simulink library "Muscles4SimScienceAB"  (R2021b)
settings: Solver=VariableStepAuto  StartTime=0.0  StopTime=10.0  RelTol=1e-3
values from neighbouring files (symbols this model uses):
  jcolor = [.4 1 .6]    [init_model_parameter.m]    (also in init_simple_main.m)
  lcolor = [.2 .6 1]    [init_model_parameter.m]    (also in init_simple_main.m; init_simple_model_parameter.m = [.5, .5 , .5])
  N = length(dataset.(fldnames{1}))    [create_timeseries.m]    (also in input_data.m = length(t); test_input_data.m = length(t))
undefined symbols (not defined in the file or in its folder): bodyparam, X, Y, Z
libraries: sm_lib x21, $bdroot x9, Library_mtu_simulink x4, nesl_utility x3
settings Model: Creator=Strel  LastModifiedBy=Strel

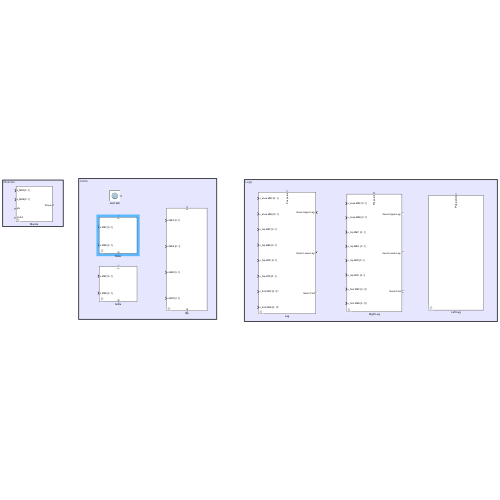
[thumbnail: Simulink's stored preview of the top-level diagram]
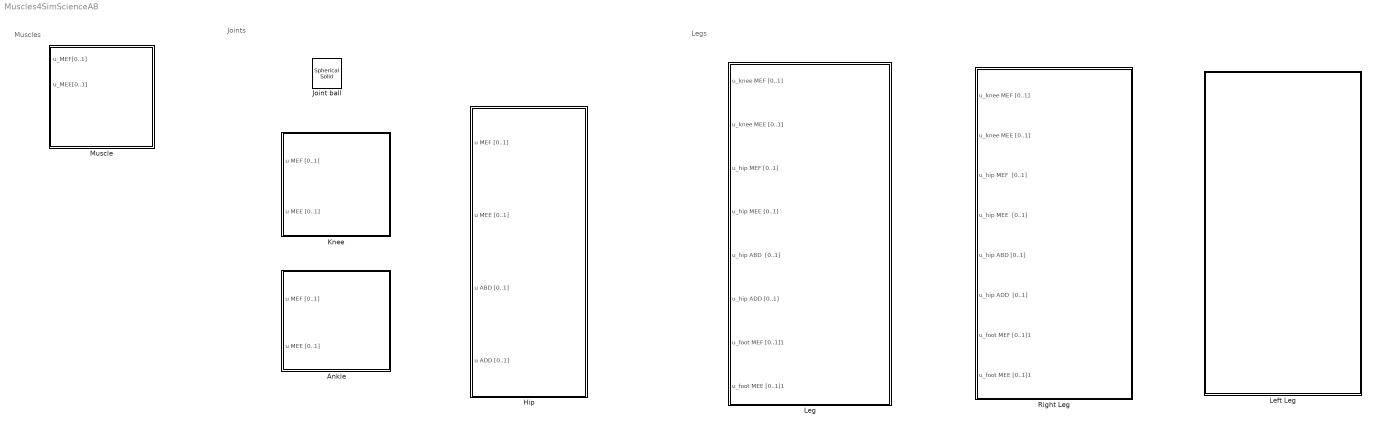
== system Muscles4SimScienceAB ==
  note: Muscles
  note: Legs
  note: Joints
  Ankle : Subsystem  mask{minlim=0, maxlim=0, stiffness=0, damping=0}
      settings: PortSchema="{\"entries\":[{\"content\":{\"sides\":[{\"content\":{\"connectorIds\":[\"In1\",\"In2\"]},\"type\":\"ConnectorPlacement.EquallySpacedRectSide\",\"uuid\":\"96b1b743-5705-4ec0-abfd-bdeea3d69127\"},{\"content\":{\"connectorIds\":[],\"side\":\"RIGHT\"},\"type\":\"ConnectorPlacement.EquallySpacedRectSide\",\"uuid\":\"b3b1b644-d2fe-42fd-b3a0-cbeacae3e2ea\"},{\"content\":{\"connectorIds\":[\"LConn1\"],\"side\":\"TOP\"},\"type\":\"ConnectorPlacement.EquallySpacedRectSide\",\"uuid\":\"6588cc9c-075c-4f00-8cf7-0671acb35c7c\"},{\"content\":{\"connectorIds\":[\"RConn1\"],\"side\":\"BOTTOM\"},\"type\":\"ConnectorPlacement.EquallySpacedRectSide\",\"uuid\":\"1f17b914-0342-4251-8355-6f738c5be59c\"}]},\"type\":\"ConnectorPlacement.EquallySpacedConnector\",\"uuid\":\"9665cf7e-0d90-4f65-9e3e-57dbf89b4304\"}],\"packageUris\":[\"http://schema.mathworks.com/mf0/Connector/R2020b\"],\"version\":\"1.0\"}"
  Hip : Subsystem  mask{minlim_x=0, maxlim_x=0, minlim_y=0, maxlim_y=0, stiffness=0, damping=0}
      settings: PortSchema="{\"entries\":[{\"content\":{\"sides\":[{\"content\":{\"connectorIds\":[\"In1\",\"In2\",\"In3\",\"In4\"]},\"type\":\"ConnectorPlacement.EquallySpacedRectSide\",\"uuid\":\"41193043-8a27-4363-8898-1f9e881d08b1\"},{\"content\":{\"connectorIds\":[],\"side\":\"RIGHT\"},\"type\":\"ConnectorPlacement.EquallySpacedRectSide\",\"uuid\":\"5a179196-4a66-423b-80c7-02c9aceed262\"},{\"content\":{\"connectorIds\":[\"LConn1\"],\"side\":\"TOP\"},\"type\":\"ConnectorPlacement.EquallySpacedRectSide\",\"uuid\":\"db447b50-73cc-4af2-8c9c-28a9801561ff\"},{\"content\":{\"connectorIds\":[\"RConn1\"],\"side\":\"BOTTOM\"},\"type\":\"ConnectorPlacement.EquallySpacedRectSide\",\"uuid\":\"bc7ed954-e11d-4420-941c-b14a31097b3c\"}]},\"type\":\"ConnectorPlacement.EquallySpacedConnector\",\"uuid\":\"a73193d2-090f-471b-ad63-2ab894437460\"}],\"packageUris\":[\"http://schema.mathworks.com/mf0/Connector/R2020b\"],\"version\":\"1.0\"}"
  Joint ball : sm_lib/Body Elements/Spherical Solid  GraphicAmbientColor=[0.15 0.15 0.15 1.0]  BasedOnType=Mass  CenterOfMass=[0 0 0]  CenterOfMassUnits=m  GraphicDiffuseColor=[1.0 1.0 0.2]  Density=1000  DensityUnits=kg/m^3  DoExposeReferenceFrame=on  GraphicEmissiveColor=[0.0 0.0 0.0 1.0]  ExportEntireGeometry=off  SerializedExposedGeometries=<ExposedGeometries/>  SerializedFrames=<Frames/>  MarkerShape=Sphere  MarkerSize=10  GraphicType=FromGeometry  InertiaType=CalculateFromGeometry  Mass=0  MassUnits=kg  MomentsOfInertia=[1 1 1]  MomentsOfInertiaUnits=kg*m^2  GraphicOpacity=1.0  ProductsOfInertia=[0 0 0]  ProductsOfInertiaUnits=kg*m^2  GraphicShininess=75  GraphicSpecularColor=[0.5 0.5 0.5 1.0]  SphereRadius=bodyparam.size.jointballs  SphereRadiusUnits=m  GraphicVisPropType=SimpleVisualProperties
  Knee : Subsystem  mask{maxlim=0, minlim=0, stiffness=0, damping=0}
      settings: PortSchema="{\"entries\":[{\"content\":{\"sides\":[{\"content\":{\"connectorIds\":[\"In1\",\"In2\"]},\"type\":\"ConnectorPlacement.EquallySpacedRectSide\",\"uuid\":\"41193043-8a27-4363-8898-1f9e881d08b1\"},{\"content\":{\"connectorIds\":[],\"side\":\"RIGHT\"},\"type\":\"ConnectorPlacement.EquallySpacedRectSide\",\"uuid\":\"5a179196-4a66-423b-80c7-02c9aceed262\"},{\"content\":{\"connectorIds\":[\"LConn1\"],\"side\":\"TOP\"},\"type\":\"ConnectorPlacement.EquallySpacedRectSide\",\"uuid\":\"db447b50-73cc-4af2-8c9c-28a9801561ff\"},{\"content\":{\"connectorIds\":[\"RConn1\"],\"side\":\"BOTTOM\"},\"type\":\"ConnectorPlacement.EquallySpacedRectSide\",\"uuid\":\"bc7ed954-e11d-4420-941c-b14a31097b3c\"}]},\"type\":\"ConnectorPlacement.EquallySpacedConnector\",\"uuid\":\"a73193d2-090f-471b-ad63-2ab894437460\"}],\"packageUris\":[\"http://schema.mathworks.com/mf0/Connector/R2020b\"],\"version\":\"1.0\"}"
  Left Leg : Subsystem  mask{pos=bodyparam.position.left, sp=bodyparam.sp.left}
      mask prompts: pos "Position"; sp "Center of Mass"
      settings: PortSchema="{\"entries\":[{\"content\":{\"sides\":[{\"content\":{\"connectorIds\":[]},\"type\":\"ConnectorPlacement.EquallySpacedRectSide\",\"uuid\":\"83ecb678-3ef8-433f-8d5c-ab0d2505f36e\"},{\"content\":{\"connectorIds\":[],\"side\":\"RIGHT\"},\"type\":\"ConnectorPlacement.EquallySpacedRectSide\",\"uuid\":\"d8e24638-d682-4ec3-8d5e-a9f0648ccc2e\"},{\"content\":{\"connectorIds\":[\"LConn1\"],\"side\":\"TOP\"},\"type\":\"ConnectorPlacement.EquallySpacedRectSide\",\"uuid\":\"3cc5390e-ac28-4512-8909-8c109732ea75\"}]},\"type\":\"ConnectorPlacement.EquallySpacedConnector\",\"uuid\":\"7489c74b-9d79-4343-b8bc-4ccd280d7c44\"}],\"packageUris\":[\"http://schema.mathworks.com/mf0/Connector/R2020b\"],\"version\":\"1.0\"}"
  Leg : Subsystem  mask{size=bodyparam.size, pos=bodyparam.position, weight=bodyparam.weight, sp=bodyparam.sp, maxlim=bodyparam.maxlim, minlim=bodyparam.minlim, stiffness=bodyparam.stiffness, damping=bodyparam.damping, jcolor=jcolor, lcolor=lcolor}
      mask prompts: pos "Position"; sp "Center of mass"; jcolor "Joint Color"; lcolor "Leg Color"
      settings: PortSchema="{\"entries\":[{\"content\":{\"sides\":[{\"content\":{\"connectorIds\":[\"In1\",\"In2\",\"In3\",\"In4\",\"In5\",\"In6\",\"In7\",\"In8\"]},\"type\":\"ConnectorPlacement.EquallySpacedRectSide\",\"uuid\":\"047c7818-584d-43bc-9ac6-0cf7022720ad\"},{\"content\":{\"connectorIds\":[\"RConn1\",\"RConn2\",\"RConn3\"],\"side\":\"RIGHT\"},\"type\":\"ConnectorPlacement.EquallySpacedRectSide\",\"uuid\":\"5ae6b5e3-6d8b-484f-b2c6-d9c9ef2af35a\"},{\"content\":{\"connectorIds\":[\"LConn1\"],\"side\":\"TOP\"},\"type\":\"ConnectorPlacement.EquallySpacedRectSide\",\"uuid\":\"10998751-961f-47ac-ace7-fed01c97684e\"}]},\"type\":\"ConnectorPlacement.EquallySpacedConnector\",\"uuid\":\"80eaa50d-578f-4e76-a7ef-cf0f1326b1e3\"}],\"packageUris\":[\"http://schema.mathworks.com/mf0/Connector/R2020b\"],\"version\":\"1.0\"}"
  Muscle : Subsystem  mask{Param_Mus_MEF=0, Param_Mus_MEE=0, r=0}
      mask prompts: r "Leverage"
  Right Leg : Subsystem  mask{pos=bodyparam.position.right, sp=bodyparam.sp.right}
      mask prompts: pos "Position"; sp "Center of Mass"
      settings: PortSchema="{\"entries\":[{\"content\":{\"sides\":[{\"content\":{\"connectorIds\":[\"In1\",\"In2\",\"In3\",\"In4\",\"In5\",\"In6\",\"In7\",\"In8\"]},\"type\":\"ConnectorPlacement.EquallySpacedRectSide\",\"uuid\":\"83ecb678-3ef8-433f-8d5c-ab0d2505f36e\"},{\"content\":{\"connectorIds\":[\"RConn1\",\"RConn2\",\"RConn3\"],\"side\":\"RIGHT\"},\"type\":\"ConnectorPlacement.EquallySpacedRectSide\",\"uuid\":\"d8e24638-d682-4ec3-8d5e-a9f0648ccc2e\"},{\"content\":{\"connectorIds\":[\"LConn1\"],\"side\":\"TOP\"},\"type\":\"ConnectorPlacement.EquallySpacedRectSide\",\"uuid\":\"3cc5390e-ac28-4512-8909-8c109732ea75\"}]},\"type\":\"ConnectorPlacement.EquallySpacedConnector\",\"uuid\":\"7489c74b-9d79-4343-b8bc-4ccd280d7c44\"}],\"packageUris\":[\"http://schema.mathworks.com/mf0/Connector/R2020b\"],\"version\":\"1.0\"}"

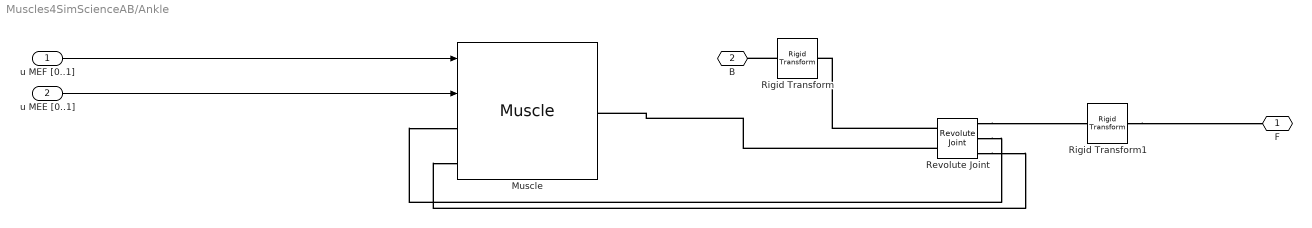
== system Muscles4SimScienceAB/Ankle ==
  u MEF [0..1] : Inport
  u MEE [0..1] : Inport  Port=2
  Muscle : $bdroot/Muscle  Param_Mus_MEF=Param_Mus_MEF_knee  Param_Mus_MEE=Param_Mus_MEE_knee  r=bodyparam.r.foot
  Revolute Joint : sm_lib/Joints/Revolute Joint  JointMode=Normal  SenseConstraintForce=off  SenseConstraintForceX=off  SenseConstraintForceY=off  SenseConstraintForceZ=off  SenseConstraintTorque=off  SenseConstraintTorqueX=off  SenseConstraintTorqueY=off  SenseConstraintTorqueZ=off  SenseTotalForce=off  SenseTotalForceX=off  SenseTotalForceY=off  SenseTotalForceZ=off  SenseTotalTorque=off  SenseTotalTorqueX=off  SenseTotalTorqueY=off  SenseTotalTorqueZ=off  CompositeWrenchDir=FollowerOnBase  CompositeWrenchFrame=BaseFrame  EquilibriumPosition=0  EquilibriumPositionUnits=deg  SpringStiffness=0  SpringStiffnessUnits=N*m/deg  DampingCoefficient=0  DampingCoefficientUnits=N*m/(deg/s)  TorqueActuationMode=InputTorque  MotionActuationMode=ComputedMotion  SensePosition=on  SenseVelocity=on  SenseAcceleration=off  SenseTorqueForce=off  SenseLowerLimitTorqueForce=off  SenseUpperLimitTorqueForce=off  LowerLimitSpecify=on  LowerLimitBound=minlim  LowerLimitBoundUnits=deg  LowerLimitStiffness=stiffness  LowerLimitStiffnessUnits=N*m/deg  LowerLimitDamping=damping  LowerLimitDampingUnits=N*m/(deg/s)  LowerLimitTransitionRegionWidth=0.1  LowerLimitTransitionRegionWidthUnits=deg  UpperLimitSpecify=on  UpperLimitBound=maxlim  UpperLimitBoundUnits=deg  UpperLimitStiffness=stiffness  UpperLimitStiffnessUnits=N*m/deg  UpperLimitDamping=damping  UpperLimitDampingUnits=N*m/(deg/s)  UpperLimitTransitionRegionWidth=0.1  UpperLimitTransitionRegionWidthUnits=deg  PositionTargetSpecify=off  PositionTargetPriority=High  PositionTargetValue=0  PositionTargetValueUnits=deg  VelocityTargetSpecify=off  VelocityTargetPriority=High  VelocityTargetValue=0  VelocityTargetValueUnits=deg/s
  Rigid Transform : sm_lib/Frames and Transforms/Rigid Transform  TranslationMethod=None  TranslationStandardOffset=0  TranslationLengthUnit=m  TranslationStandardAxis=+Z  TranslationCartesianOffset=[0 0 0]  TranslationROffset=0  TranslationROffsetUnits=m  TranslationZOffset=0  TranslationZOffsetUnits=m  TranslationThetaOffset=0  TranslationThetaOffsetUnits=deg  RotationMethod=StandardAxis  RotationAngleUnits=deg  RotationStandardAxis=+X  RotationAngle=-90  RotationArbitraryAxis=[0 0 1]  FollAlignAxisA=+X  BaseAlignAxisA=+Y  FollAlignAxisB=+Y  BaseAlignAxisB=+Z  RotationSequenceAxes=FollowerAxes  RotationSequence=XYX  RotationSequenceAngles=[0 0 0]  RotationSequenceAnglesUnits=deg  RotationMatrix=[1 0 0; 0 1 0; 0 0 1]
  Rigid Transform1 : sm_lib/Frames and Transforms/Rigid Transform  TranslationMethod=None  TranslationStandardOffset=0  TranslationLengthUnit=m  TranslationStandardAxis=+Z  TranslationCartesianOffset=[0 0 0]  TranslationROffset=0  TranslationROffsetUnits=m  TranslationZOffset=0  TranslationZOffsetUnits=m  TranslationThetaOffset=0  TranslationThetaOffsetUnits=deg  RotationMethod=StandardAxis  RotationAngleUnits=deg  RotationStandardAxis=+X  RotationAngle=90  RotationArbitraryAxis=[0 0 1]  FollAlignAxisA=+X  BaseAlignAxisA=+Y  FollAlignAxisB=+Y  BaseAlignAxisB=+Z  RotationSequenceAxes=FollowerAxes  RotationSequence=XYX  RotationSequenceAngles=[0 0 0]  RotationSequenceAnglesUnits=deg  RotationMatrix=[1 0 0; 0 1 0; 0 0 1]
  F : PMIOPort  Side=Left
  B : PMIOPort  Port=2  Side=Right
  wires:
  u MEE [0..1]/1 -> Muscle/2
  u MEF [0..1]/1 -> Muscle/1
  connections:
  Rigid Transform/LConn1 -- B/RConn1
  Revolute Joint/RConn1 -- Rigid Transform1/LConn1
  Revolute Joint/LConn2 -- Muscle/RConn1
  Revolute Joint/RConn3 -- Muscle/LConn2
  Revolute Joint/LConn1 -- Rigid Transform/RConn1
  Rigid Transform1/RConn1 -- F/RConn1
  Revolute Joint/RConn2 -- Muscle/LConn1

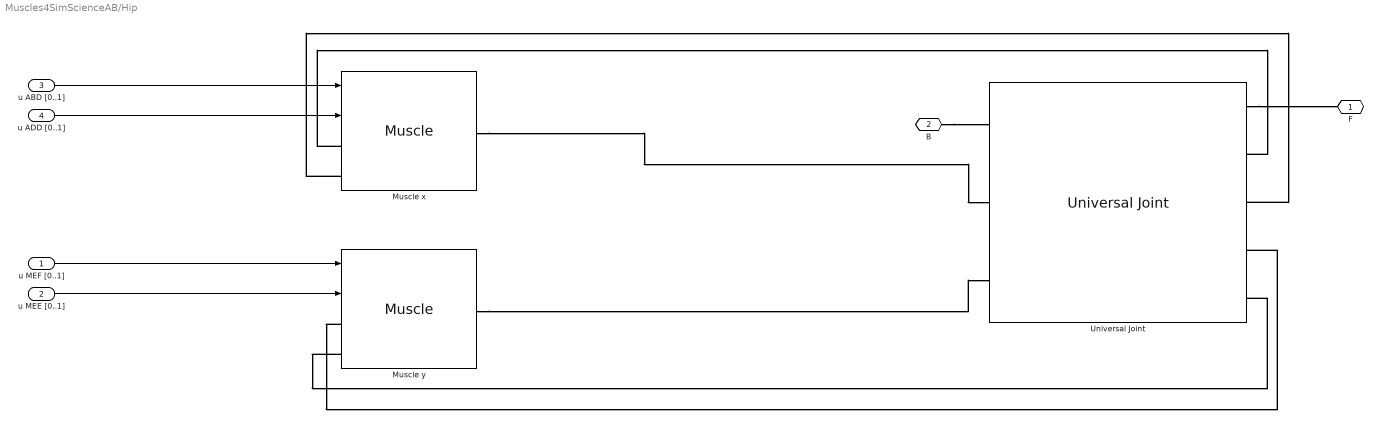
== system Muscles4SimScienceAB/Hip ==
  u MEF [0..1] : Inport
  u MEE [0..1] : Inport  Port=2
  u ABD [0..1] : Inport  Port=3
  u ADD [0..1] : Inport  Port=4
  Muscle x : $bdroot/Muscle  Param_Mus_MEF=Param_Mus_MEF_hip  Param_Mus_MEE=Param_Mus_MEE_hip  r=bodyparam.r.hip.ef
  Muscle y : $bdroot/Muscle  Param_Mus_MEF=Param_Mus_ABD_hip  Param_Mus_MEE=Param_Mus_ADD_hip  r=bodyparam.r.hip.abd
  Universal Joint : sm_lib/Joints/Universal Joint  JointMode=Normal  SenseConstraintForce=off  SenseConstraintForceX=off  SenseConstraintForceY=off  SenseConstraintForceZ=off  SenseConstraintTorque=off  SenseConstraintTorqueX=off  SenseConstraintTorqueY=off  SenseConstraintTorqueZ=off  SenseTotalForce=off  SenseTotalForceX=off  SenseTotalForceY=off  SenseTotalForceZ=off  SenseTotalTorque=off  SenseTotalTorqueX=off  SenseTotalTorqueY=off  SenseTotalTorqueZ=off  CompositeWrenchDir=FollowerOnBase  CompositeWrenchFrame=BaseFrame  RxEquilibriumPosition=0  RxEquilibriumPositionUnits=deg  RxSpringStiffness=0  RxSpringStiffnessUnits=N*m/deg  RxDampingCoefficient=0  RxDampingCoefficientUnits=N*m/(deg/s)  RxTorqueActuationMode=InputTorque  RxMotionActuationMode=ComputedMotion  RxSensePosition=on  RxSenseVelocity=on  RxSenseAcceleration=off  RxSenseTorqueForce=off  RxSenseLowerLimitTorqueForce=off  RxSenseUpperLimitTorqueForce=off  RxLowerLimitSpecify=on  RxLowerLimitBound=minlim_x  RxLowerLimitBoundUnits=deg  RxLowerLimitStiffness=stiffness  RxLowerLimitStiffnessUnits=N*m/deg  RxLowerLimitDamping=damping  RxLowerLimitDampingUnits=N*m/(deg/s)  RxLowerLimitTransitionRegionWidth=0.1  RxLowerLimitTransitionRegionWidthUnits=deg  RxUpperLimitSpecify=on  RxUpperLimitBound=maxlim_x  RxUpperLimitBoundUnits=deg  RxUpperLimitStiffness=stiffness  RxUpperLimitStiffnessUnits=N*m/deg  RxUpperLimitDamping=damping  RxUpperLimitDampingUnits=N*m*s/deg  RxUpperLimitTransitionRegionWidth=0.1  RxUpperLimitTransitionRegionWidthUnits=deg  RxPositionTargetSpecify=off  RxPositionTargetPriority=High  RxPositionTargetValue=0  RxPositionTargetValueUnits=deg  RxVelocityTargetSpecify=off  RxVelocityTargetPriority=High  RxVelocityTargetValue=0  RxVelocityTargetValueUnits=deg/s  RyEquilibriumPosition=0  RyEquilibriumPositionUnits=deg  RySpringStiffness=0  RySpringStiffnessUnits=N*m/deg  RyDampingCoefficient=0  RyDampingCoefficientUnits=N*m/(deg/s)  RyTorqueActuationMode=InputTorque  RyMotionActuationMode=ComputedMotion  RySensePosition=on  RySenseVelocity=on  RySenseAcceleration=off  RySenseTorqueForce=off  RySenseLowerLimitTorqueForce=off  RySenseUpperLimitTorqueForce=off  RyLowerLimitSpecify=on  RyLowerLimitBound=minlim_y  RyLowerLimitBoundUnits=deg  RyLowerLimitStiffness=stiffness  RyLowerLimitStiffnessUnits=N*m/deg  RyLowerLimitDamping=damping  RyLowerLimitDampingUnits=N*m/(deg/s)  RyLowerLimitTransitionRegionWidth=0.1  RyLowerLimitTransitionRegionWidthUnits=deg  RyUpperLimitSpecify=on  RyUpperLimitBound=maxlim_y  RyUpperLimitBoundUnits=deg  RyUpperLimitStiffness=stiffness  RyUpperLimitStiffnessUnits=N*m/deg  RyUpperLimitDamping=damping  RyUpperLimitDampingUnits=N*m/(deg/s)  RyUpperLimitTransitionRegionWidth=0.1  RyUpperLimitTransitionRegionWidthUnits=deg  RyPositionTargetSpecify=off  RyPositionTargetPriority=High  RyPositionTargetValue=0  RyPositionTargetValueUnits=deg  RyVelocityTargetSpecify=off  RyVelocityTargetPriority=High  RyVelocityTargetValue=0  RyVelocityTargetValueUnits=deg/s
  F : PMIOPort  Side=Left
  B : PMIOPort  Port=2  Side=Right
  wires:
  u ABD [0..1]/1 -> Muscle x/1
  u ADD [0..1]/1 -> Muscle x/2
  u MEF [0..1]/1 -> Muscle y/1
  u MEE [0..1]/1 -> Muscle y/2
  connections:
  Muscle x/RConn1 -- Universal Joint/LConn2
  Muscle y/RConn1 -- Universal Joint/LConn3
  B/RConn1 -- Universal Joint/LConn1
  Muscle x/LConn1 -- Universal Joint/RConn2
  Universal Joint/RConn1 -- F/RConn1
  Muscle x/LConn2 -- Universal Joint/RConn3
  Muscle y/LConn1 -- Universal Joint/RConn4
  Muscle y/LConn2 -- Universal Joint/RConn5

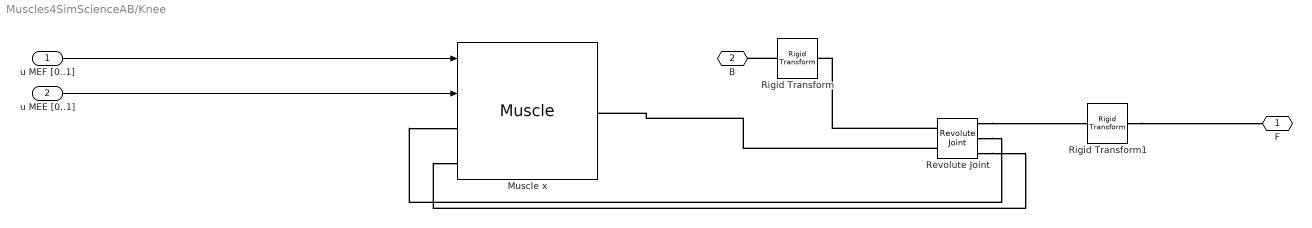
== system Muscles4SimScienceAB/Knee ==
  u MEF [0..1] : Inport
  u MEE [0..1] : Inport  Port=2
  Muscle x : $bdroot/Muscle  Param_Mus_MEF=Param_Mus_MEF_knee  Param_Mus_MEE=Param_Mus_MEE_knee  r=bodyparam.r.knee
  Revolute Joint : sm_lib/Joints/Revolute Joint  JointMode=Normal  SenseConstraintForce=off  SenseConstraintForceX=off  SenseConstraintForceY=off  SenseConstraintForceZ=off  SenseConstraintTorque=off  SenseConstraintTorqueX=off  SenseConstraintTorqueY=off  SenseConstraintTorqueZ=off  SenseTotalForce=off  SenseTotalForceX=off  SenseTotalForceY=off  SenseTotalForceZ=off  SenseTotalTorque=off  SenseTotalTorqueX=off  SenseTotalTorqueY=off  SenseTotalTorqueZ=off  CompositeWrenchDir=FollowerOnBase  CompositeWrenchFrame=BaseFrame  EquilibriumPosition=0  EquilibriumPositionUnits=deg  SpringStiffness=0  SpringStiffnessUnits=N*m/deg  DampingCoefficient=0  DampingCoefficientUnits=N*m/(deg/s)  TorqueActuationMode=InputTorque  MotionActuationMode=ComputedMotion  SensePosition=on  SenseVelocity=on  SenseAcceleration=off  SenseTorqueForce=off  SenseLowerLimitTorqueForce=off  SenseUpperLimitTorqueForce=off  LowerLimitSpecify=on  LowerLimitBound=minlim  LowerLimitBoundUnits=deg  LowerLimitStiffness=stiffness  LowerLimitStiffnessUnits=N*m/deg  LowerLimitDamping=damping  LowerLimitDampingUnits=N*m/(deg/s)  LowerLimitTransitionRegionWidth=0.1  LowerLimitTransitionRegionWidthUnits=deg  UpperLimitSpecify=on  UpperLimitBound=maxlim  UpperLimitBoundUnits=deg  UpperLimitStiffness=stiffness  UpperLimitStiffnessUnits=N*m/deg  UpperLimitDamping=damping  UpperLimitDampingUnits=N*m/(deg/s)  UpperLimitTransitionRegionWidth=0.1  UpperLimitTransitionRegionWidthUnits=deg  PositionTargetSpecify=off  PositionTargetPriority=High  PositionTargetValue=0  PositionTargetValueUnits=deg  VelocityTargetSpecify=off  VelocityTargetPriority=High  VelocityTargetValue=0  VelocityTargetValueUnits=deg/s
  Rigid Transform : sm_lib/Frames and Transforms/Rigid Transform  TranslationMethod=None  TranslationStandardOffset=0  TranslationLengthUnit=m  TranslationStandardAxis=+Z  TranslationCartesianOffset=[0 0 0]  TranslationROffset=0  TranslationROffsetUnits=m  TranslationZOffset=0  TranslationZOffsetUnits=m  TranslationThetaOffset=0  TranslationThetaOffsetUnits=deg  RotationMethod=StandardAxis  RotationAngleUnits=deg  RotationStandardAxis=+X  RotationAngle=-90  RotationArbitraryAxis=[0 0 1]  FollAlignAxisA=+X  BaseAlignAxisA=+Y  FollAlignAxisB=+Y  BaseAlignAxisB=+Z  RotationSequenceAxes=FollowerAxes  RotationSequence=XYX  RotationSequenceAngles=[0 0 0]  RotationSequenceAnglesUnits=deg  RotationMatrix=[1 0 0; 0 1 0; 0 0 1]
  Rigid Transform1 : sm_lib/Frames and Transforms/Rigid Transform  TranslationMethod=None  TranslationStandardOffset=0  TranslationLengthUnit=m  TranslationStandardAxis=+Z  TranslationCartesianOffset=[0 0 0]  TranslationROffset=0  TranslationROffsetUnits=m  TranslationZOffset=0  TranslationZOffsetUnits=m  TranslationThetaOffset=0  TranslationThetaOffsetUnits=deg  RotationMethod=StandardAxis  RotationAngleUnits=deg  RotationStandardAxis=+X  RotationAngle=90  RotationArbitraryAxis=[0 0 1]  FollAlignAxisA=+X  BaseAlignAxisA=+Y  FollAlignAxisB=+Y  BaseAlignAxisB=+Z  RotationSequenceAxes=FollowerAxes  RotationSequence=XYX  RotationSequenceAngles=[0 0 0]  RotationSequenceAnglesUnits=deg  RotationMatrix=[1 0 0; 0 1 0; 0 0 1]
  F : PMIOPort  Side=Left
  B : PMIOPort  Port=2  Side=Right
  wires:
  u MEE [0..1]/1 -> Muscle x/2
  u MEF [0..1]/1 -> Muscle x/1
  connections:
  Revolute Joint/LConn1 -- Rigid Transform/RConn1
  Revolute Joint/LConn2 -- Muscle x/RConn1
  Rigid Transform1/RConn1 -- F/RConn1
  Revolute Joint/RConn2 -- Muscle x/LConn1
  Revolute Joint/RConn3 -- Muscle x/LConn2
  Rigid Transform/LConn1 -- B/RConn1
  Revolute Joint/RConn1 -- Rigid Transform1/LConn1

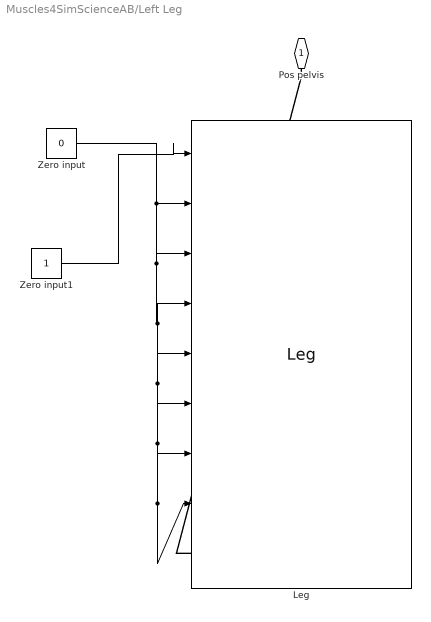
== system Muscles4SimScienceAB/Left Leg ==
  Leg : $bdroot/Leg  size=bodyparam.size  pos=pos  weight=bodyparam.weight  sp=sp  maxlim=bodyparam.maxlim  minlim=bodyparam.minlim  stiffness=bodyparam.stiffness  damping=bodyparam.damping  jcolor=jcolor  lcolor=lcolor
      link override Upper Leg Right/Hip: minlim_x=minlim.hip.ef  maxlim_x=maxlim.hip.ef  minlim_y=minlim.hip.abd  maxlim_y=maxlim.hip.abd  stiffness=stiffness.hip  damping=damping.hip
  Zero input : Constant  Value=0
  Zero input1 : Constant
  Pos pelvis : PMIOPort  Side=Left
  wires:
  Zero input/1 -> Leg/2, Leg/3, Leg/4, Leg/5, Leg/6, Leg/7, Leg/8
  Zero input1/1 -> Leg/1
  connections:
  Leg/LConn1 -- Pos pelvis/RConn1

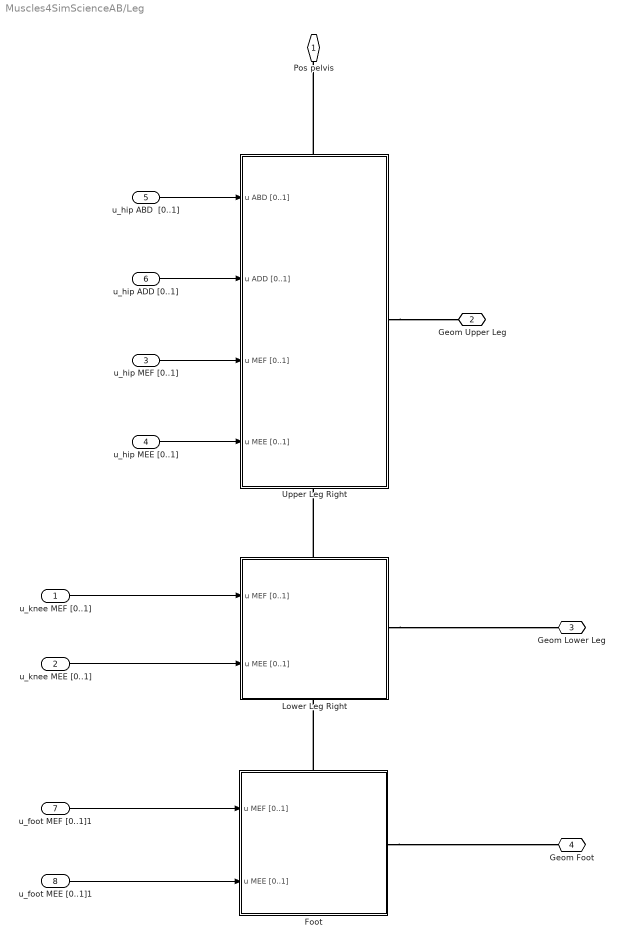
== system Muscles4SimScienceAB/Leg ==
  u_knee MEF [0..1] : Inport
  u_knee MEE [0..1] : Inport  Port=2
  u_hip MEF [0..1] : Inport  Port=3
  u_hip MEE [0..1] : Inport  Port=4
  u_hip ABD  [0..1] : Inport  Port=5
  u_hip ADD [0..1] : Inport  Port=6
  u_foot MEF [0..1]1 : Inport  Port=7
  u_foot MEE [0..1]1 : Inport  Port=8
  Foot : Subsystem
      settings: PortSchema="{\"entries\":[{\"content\":{\"sides\":[{\"content\":{\"connectorIds\":[]},\"type\":\"ConnectorPlacement.EquallySpacedRectSide\",\"uuid\":\"d033d68b-6c1a-4130-88bc-96923c9206ae\"},{\"content\":{\"connectorIds\":[\"RConn1\"],\"side\":\"RIGHT\"},\"type\":\"ConnectorPlacement.EquallySpacedRectSide\",\"uuid\":\"aebe2891-e167-481b-874d-322841d1d85d\"},{\"content\":{\"connectorIds\":[\"In1\",\"In2\"],\"side\":\"TOP\"},\"type\":\"ConnectorPlacement.EquallySpacedRectSide\",\"uuid\":\"02ffbb51-7d33-4a0b-abb1-a48a3de38eb7\"},{\"content\":{\"connectorIds\":[\"RConn2\"],\"side\":\"BOTTOM\"},\"type\":\"ConnectorPlacement.EquallySpacedRectSide\",\"uuid\":\"55de7e85-58cc-4707-ad35-b95b4479c51b\"}]},\"type\":\"ConnectorPlacement.EquallySpacedConnector\",\"uuid\":\"eef9a049-18d9-4a2f-a245-6d7e22390965\"}],\"packageUris\":[\"http://schema.mathworks.com/mf0/Connector/R2020b\"],\"version\":\"1.0\"}"
  Lower Leg Right : Subsystem
      settings: PortSchema="{\"entries\":[{\"content\":{\"sides\":[{\"content\":{\"connectorIds\":[\"LConn1\"]},\"type\":\"ConnectorPlacement.EquallySpacedRectSide\",\"uuid\":\"81fd97e6-5a65-4706-89fa-4293b691d4da\"},{\"content\":{\"connectorIds\":[\"RConn1\"],\"side\":\"RIGHT\"},\"type\":\"ConnectorPlacement.EquallySpacedRectSide\",\"uuid\":\"97541aff-136c-4e86-8809-6e6381c3329c\"},{\"content\":{\"connectorIds\":[\"In1\",\"In2\"],\"side\":\"TOP\"},\"type\":\"ConnectorPlacement.EquallySpacedRectSide\",\"uuid\":\"ce41e290-bfc8-4dfc-8c5e-525607ac3665\"},{\"content\":{\"connectorIds\":[\"RConn2\"],\"side\":\"BOTTOM\"},\"type\":\"ConnectorPlacement.EquallySpacedRectSide\",\"uuid\":\"f37d3c0f-447d-4b24-96cc-929e66a7279d\"}]},\"type\":\"ConnectorPlacement.EquallySpacedConnector\",\"uuid\":\"c782017f-7d61-4987-8163-b5d1e1eaf397\"}],\"packageUris\":[\"http://schema.mathworks.com/mf0/Connector/R2020b\"],\"version\":\"1.0\"}"
  Upper Leg Right : Subsystem
      settings: PortSchema="{\"entries\":[{\"content\":{\"sides\":[{\"content\":{\"connectorIds\":[\"LConn1\"]},\"type\":\"ConnectorPlacement.EquallySpacedRectSide\",\"uuid\":\"81fd97e6-5a65-4706-89fa-4293b691d4da\"},{\"content\":{\"connectorIds\":[\"RConn1\"],\"side\":\"RIGHT\"},\"type\":\"ConnectorPlacement.EquallySpacedRectSide\",\"uuid\":\"97541aff-136c-4e86-8809-6e6381c3329c\"},{\"content\":{\"connectorIds\":[\"In1\",\"In2\",\"In3\",\"In4\"],\"side\":\"TOP\"},\"type\":\"ConnectorPlacement.EquallySpacedRectSide\",\"uuid\":\"ce41e290-bfc8-4dfc-8c5e-525607ac3665\"},{\"content\":{\"connectorIds\":[\"RConn2\"],\"side\":\"BOTTOM\"},\"type\":\"ConnectorPlacement.EquallySpacedRectSide\",\"uuid\":\"2db09f85-d22e-4c52-ab8b-45b3630dfd34\"}]},\"type\":\"ConnectorPlacement.EquallySpacedConnector\",\"uuid\":\"c782017f-7d61-4987-8163-b5d1e1eaf397\"}],\"packageUris\":[\"http://schema.mathworks.com/mf0/Connector/R2020b\"],\"version\":\"1.0\"}"
  Pos pelvis : PMIOPort  Side=Left
  "Geom Upper Leg " : PMIOPort  Port=2  Side=Right
  "Geom Lower Leg " : PMIOPort  Port=3  Side=Right
  Geom Foot : PMIOPort  Port=4  Side=Right
  wires:
  u_knee MEF [0..1]/1 -> Lower Leg Right/2(u MEF [0..1])
  u_knee MEE [0..1]/1 -> Lower Leg Right/1(u MEE [0..1])
  u_foot MEF [0..1]1/1 -> Foot/2(u MEF [0..1])
  u_foot MEE [0..1]1/1 -> Foot/1(u MEE [0..1])
  u_hip ADD [0..1]/1 -> Upper Leg Right/3(u ADD [0..1])
  u_hip ABD  [0..1]/1 -> Upper Leg Right/4(u ABD [0..1])
  u_hip MEF [0..1]/1 -> Upper Leg Right/2(u MEF [0..1])
  u_hip MEE [0..1]/1 -> Upper Leg Right/1(u MEE [0..1])
  connections:
  Upper Leg Right/RConn1 -- Pos pelvis/RConn1
  Upper Leg Right/RConn2 -- "Geom Upper Leg "/RConn1
  Foot/RConn1 -- Lower Leg Right/LConn1
  Lower Leg Right/RConn2 -- "Geom Lower Leg "/RConn1
  Lower Leg Right/RConn1 -- Upper Leg Right/LConn1
  Foot/RConn2 -- Geom Foot/RConn1

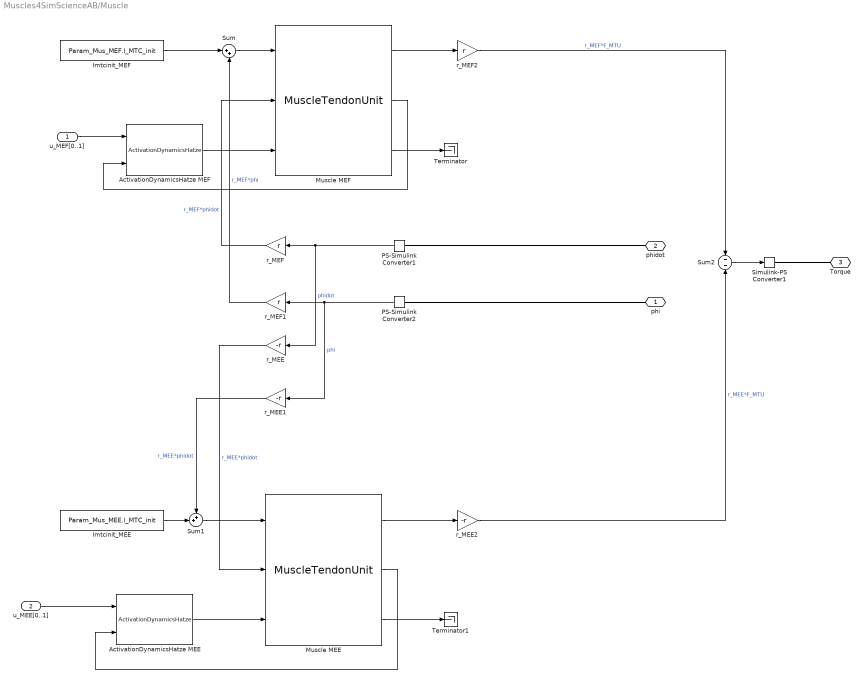
== system Muscles4SimScienceAB/Muscle ==
  u_MEF[0..1] : Inport
  u_MEE[0..1] : Inport  Port=2
  ActivationDynamicsHatze MEE : Library_mtu_simulink/ActivationDynamicsHatze  Act_Param=Param_Mus_MEE.ActDyn  Mus_Param=Param_Mus_MEE
  ActivationDynamicsHatze MEF : Library_mtu_simulink/ActivationDynamicsHatze  Act_Param=Param_Mus_MEF.ActDyn  Mus_Param=Param_Mus_MEF
  Imtcinit_MEE : Constant  Value=Param_Mus_MEE.l_MTC_init
  Imtcinit_MEF : Constant  Value=Param_Mus_MEF.l_MTC_init
  Muscle MEE : Library_mtu_simulink/MuscleTendonUnit  Mus_Param=Param_Mus_MEE
  Muscle MEF : Library_mtu_simulink/MuscleTendonUnit  Mus_Param=Param_Mus_MEF
  PS-Simulink Converter1 : nesl_utility/PS-Simulink Converter  PhysicalDomain=network_engine_domain  SubClassName=ps_output  LeftPortType=input  RightPortType=output  PseudoPeriodic=off  Frequencies=[]  Unit=inherit  AffineConversion=off
      settings: SourceProductBaseCode=PW,SS
  PS-Simulink Converter2 : nesl_utility/PS-Simulink Converter  PhysicalDomain=network_engine_domain  SubClassName=ps_output  LeftPortType=input  RightPortType=output  PseudoPeriodic=off  Frequencies=[]  Unit=inherit  AffineConversion=off
      settings: SourceProductBaseCode=PW,SS
  Simulink-PS Converter1 : nesl_utility/Simulink-PS Converter  PhysicalDomain=network_engine_domain  SubClassName=ps_input  LeftPortType=input  RightPortType=output  PseudoPeriodic=off  Frequencies=[]  NoiseDistribution=none  NoiseParameters=[]  Unit=1  AffineConversion=off  FilteringAndDerivatives=provide  SimscapeFilterOrder=1  InputFilterTimeConstant=0.001  UdotUserProvided=0
      settings: SourceProductBaseCode=PW,SS
  Sum : Sum  Inputs=|++
  Sum1 : Sum  Inputs=++|
  Sum2 : Sum  Inputs=--
  Terminator : Terminator
  Terminator1 : Terminator
  r_MEE : Gain  Gain=-r
  r_MEE1 : Gain  Gain=-r
  r_MEE2 : Gain  Gain=-r
  r_MEF : Gain  Gain=r
  r_MEF1 : Gain  Gain=r
  r_MEF2 : Gain  Gain=r
  phi : PMIOPort  Side=Left
  phidot : PMIOPort  Port=2  Side=Left
  Torque : PMIOPort  Port=3  Side=Right
  wires:
  r_MEE1/1 -> Sum1/1  "r_MEE*phidot"
  ActivationDynamicsHatze MEF/1 -> Muscle MEF/3
  u_MEF[0..1]/1 -> ActivationDynamicsHatze MEF/1
  r_MEE2/1 -> Sum2/2  "r_MEE*F_MTU"
  r_MEF/1 -> Muscle MEF/2  "r_MEF*phidot"
  Sum2/1 -> Simulink-PS Converter1/1
  Muscle MEE/1 -> r_MEE2/1
  Sum1/1 -> Muscle MEE/1
  ActivationDynamicsHatze MEE/1 -> Muscle MEE/3
  u_MEE[0..1]/1 -> ActivationDynamicsHatze MEE/1
  Muscle MEE/2 -> ActivationDynamicsHatze MEE/2
  r_MEE/1 -> Muscle MEE/2  "r_MEE*phidot"
  Imtcinit_MEE/1 -> Sum1/2
  Muscle MEF/1 -> r_MEF2/1
  PS-Simulink Converter1/1 -> r_MEE/1, r_MEF/1  "phidot"
  Muscle MEF/2 -> ActivationDynamicsHatze MEF/2
  PS-Simulink Converter2/1 -> r_MEE1/1, r_MEF1/1  "phi"
  r_MEF1/1 -> Sum/2  "r_MEF*phi"
  Muscle MEF/3 -> Terminator/1
  Sum/1 -> Muscle MEF/1
  Imtcinit_MEF/1 -> Sum/1
  r_MEF2/1 -> Sum2/1  "r_MEF*F_MTU"
  Muscle MEE/3 -> Terminator1/1
  connections:
  PS-Simulink Converter1/LConn1 -- phidot/RConn1
  PS-Simulink Converter2/LConn1 -- phi/RConn1
  Torque/RConn1 -- Simulink-PS Converter1/RConn1

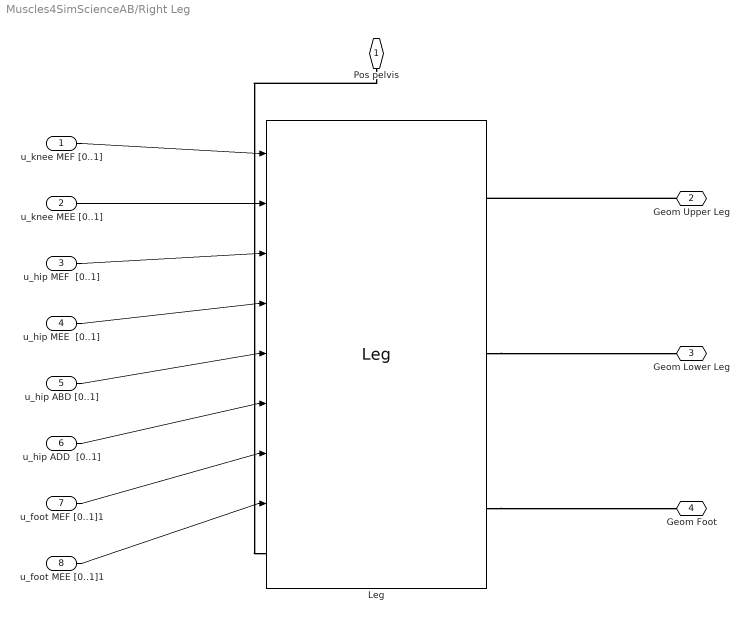
== system Muscles4SimScienceAB/Right Leg ==
  u_knee MEF [0..1] : Inport
  u_knee MEE [0..1] : Inport  Port=2
  u_hip MEF  [0..1] : Inport  Port=3
  u_hip MEE  [0..1] : Inport  Port=4
  u_hip ABD [0..1] : Inport  Port=5
  u_hip ADD  [0..1] : Inport  Port=6
  u_foot MEF [0..1]1 : Inport  Port=7
  u_foot MEE [0..1]1 : Inport  Port=8
  Leg : $bdroot/Leg  size=bodyparam.size  pos=pos  weight=bodyparam.weight  sp=sp  maxlim=bodyparam.maxlim  minlim=bodyparam.minlim  stiffness=bodyparam.stiffness  damping=bodyparam.damping  jcolor=jcolor  lcolor=lcolor
      link override Upper Leg Right/Hip: minlim_x=minlim.hip.abd  maxlim_x=maxlim.hip.abd  minlim_y=minlim.hip.ef  maxlim_y=maxlim.hip.ef  stiffness=stiffness.hip  damping=damping.hip
  Pos pelvis : PMIOPort  Side=Left
  "Geom Upper Leg " : PMIOPort  Port=2  Side=Right
  "Geom Lower Leg " : PMIOPort  Port=3  Side=Right
  Geom Foot : PMIOPort  Port=4  Side=Right
  wires:
  u_hip MEF  [0..1]/1 -> Leg/3
  u_knee MEE [0..1]/1 -> Leg/2
  u_hip ABD [0..1]/1 -> Leg/5
  u_knee MEF [0..1]/1 -> Leg/1
  u_foot MEE [0..1]1/1 -> Leg/8
  u_foot MEF [0..1]1/1 -> Leg/7
  u_hip ADD  [0..1]/1 -> Leg/6
  u_hip MEE  [0..1]/1 -> Leg/4
  connections:
  Pos pelvis/RConn1 -- Leg/LConn1
  "Geom Upper Leg "/RConn1 -- Leg/RConn1
  Leg/RConn2 -- "Geom Lower Leg "/RConn1
  Leg/RConn3 -- Geom Foot/RConn1

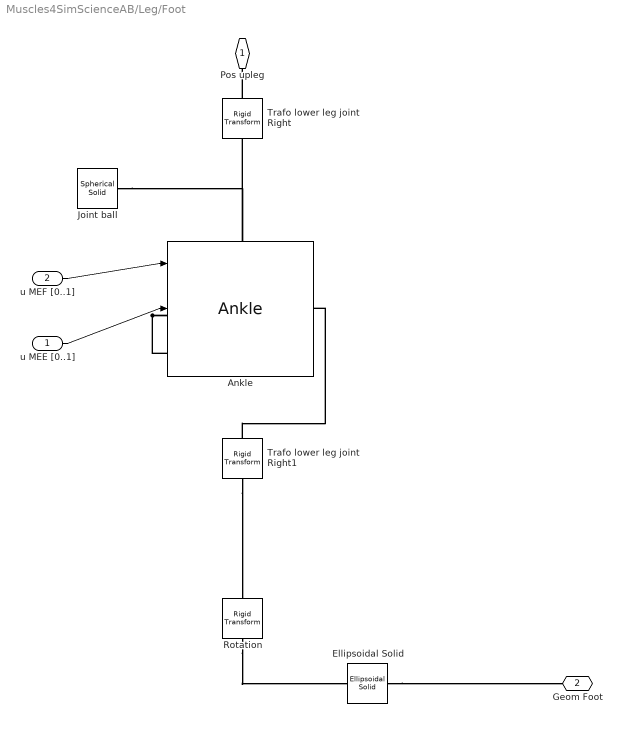
== system Muscles4SimScienceAB/Leg/Foot ==
  u MEE [0..1] : Inport
  u MEF [0..1] : Inport  Port=2
  Ankle : $bdroot/Ankle  minlim=minlim.ankle  maxlim=maxlim.ankle  stiffness=stiffness.ankle  damping=damping.ankle
  Ellipsoidal Solid : sm_lib/Body Elements/Ellipsoidal Solid  GraphicAmbientColor=[0.15 0.15 0.15 1.0]  BasedOnType=Density  CenterOfMass=[0 0 0]  CenterOfMassUnits=m  GraphicDiffuseColor=lcolor  Density=1000  DensityUnits=kg/m^3  DoExposeReferenceFrame=on  EllipsoidRadii=size.foot/2  EllipsoidRadiiUnits=m  GraphicEmissiveColor=[0.0 0.0 0.0 1.0]  ExportEntireGeometry=on  SerializedFrames=<Frames/>  MarkerShape=Sphere  MarkerSize=10  GraphicType=FromGeometry  InertiaType=CalculateFromGeometry  Mass=1  MassUnits=kg  MomentsOfInertia=[1 1 1]  MomentsOfInertiaUnits=kg*m^2  GraphicOpacity=1.0  ProductsOfInertia=[0 0 0]  ProductsOfInertiaUnits=kg*m^2  GraphicShininess=75  GraphicSpecularColor=[0.5 0.5 0.5 1.0]  GraphicVisPropType=SimpleVisualProperties
      settings: SourceProductBaseCode=MS
  Joint ball : sm_lib/Body Elements/Spherical Solid  GraphicAmbientColor=[0.15 0.15 0.15 1.0]  BasedOnType=Mass  CenterOfMass=[0 0 0]  CenterOfMassUnits=m  GraphicDiffuseColor=jcolor  Density=1000  DensityUnits=kg/m^3  DoExposeReferenceFrame=on  GraphicEmissiveColor=[0.0 0.0 0.0 1.0]  ExportEntireGeometry=off  SerializedExposedGeometries=<ExposedGeometries/>  SerializedFrames=<Frames/>  MarkerShape=Sphere  MarkerSize=10  GraphicType=FromGeometry  InertiaType=CalculateFromGeometry  Mass=0  MassUnits=kg  MomentsOfInertia=[1 1 1]  MomentsOfInertiaUnits=kg*m^2  GraphicOpacity=1.0  ProductsOfInertia=[0 0 0]  ProductsOfInertiaUnits=kg*m^2  GraphicShininess=75  GraphicSpecularColor=[0.5 0.5 0.5 1.0]  SphereRadius=size.jointballs  SphereRadiusUnits=m  GraphicVisPropType=SimpleVisualProperties
  Rotation : sm_lib/Frames and Transforms/Rigid Transform  TranslationMethod=None  TranslationStandardOffset=0  TranslationLengthUnit=m  TranslationStandardAxis=+Z  TranslationCartesianOffset=[0 0 0]  TranslationROffset=0  TranslationROffsetUnits=m  TranslationZOffset=0  TranslationZOffsetUnits=m  TranslationThetaOffset=0  TranslationThetaOffsetUnits=deg  RotationMethod=StandardAxis  RotationAngleUnits=deg  RotationStandardAxis=+Y  RotationAngle=90  RotationArbitraryAxis=[0 0 1]  FollAlignAxisA=+X  BaseAlignAxisA=+Y  FollAlignAxisB=+Y  BaseAlignAxisB=+Z  RotationSequenceAxes=FollowerAxes  RotationSequence=XYX  RotationSequenceAngles=[0 0 0]  RotationSequenceAnglesUnits=deg  RotationMatrix=[1 0 0; 0 1 0; 0 0 1]
  Trafo lower leg joint Right : sm_lib/Frames and Transforms/Rigid Transform  TranslationMethod=Cartesian  TranslationStandardOffset=0  TranslationLengthUnit=m  TranslationStandardAxis=+Z  TranslationCartesianOffset=pos.foot.joint  TranslationROffset=0  TranslationROffsetUnits=m  TranslationZOffset=0  TranslationZOffsetUnits=m  TranslationThetaOffset=0  TranslationThetaOffsetUnits=deg  RotationMethod=None  RotationAngleUnits=deg  RotationStandardAxis=+Z  RotationAngle=0.0  RotationArbitraryAxis=[0 0 1]  FollAlignAxisA=+X  BaseAlignAxisA=+Y  FollAlignAxisB=+Y  BaseAlignAxisB=+Z  RotationSequenceAxes=FollowerAxes  RotationSequence=XYX  RotationSequenceAngles=[0 0 0]  RotationSequenceAnglesUnits=deg  RotationMatrix=[1 0 0; 0 1 0; 0 0 1]
  Trafo lower leg joint Right1 : sm_lib/Frames and Transforms/Rigid Transform  TranslationMethod=Cartesian  TranslationStandardOffset=0  TranslationLengthUnit=m  TranslationStandardAxis=+Z  TranslationCartesianOffset=pos.foot.item  TranslationROffset=0  TranslationROffsetUnits=m  TranslationZOffset=0  TranslationZOffsetUnits=m  TranslationThetaOffset=0  TranslationThetaOffsetUnits=deg  RotationMethod=None  RotationAngleUnits=deg  RotationStandardAxis=+Z  RotationAngle=0.0  RotationArbitraryAxis=[0 0 1]  FollAlignAxisA=+X  BaseAlignAxisA=+Y  FollAlignAxisB=+Y  BaseAlignAxisB=+Z  RotationSequenceAxes=FollowerAxes  RotationSequence=XYX  RotationSequenceAngles=[0 0 0]  RotationSequenceAnglesUnits=deg  RotationMatrix=[1 0 0; 0 1 0; 0 0 1]
  Pos upleg : PMIOPort  Side=Right
  Geom Foot : PMIOPort  Port=2  Side=Right
  wires:
  u MEE [0..1]/1 -> Ankle/2
  u MEF [0..1]/1 -> Ankle/1
  connections:
  Trafo lower leg joint Right/LConn1 -- Pos upleg/RConn1
  Ankle/LConn1 -- Joint ball/RConn1 -- Trafo lower leg joint Right/RConn1
  Rotation/RConn1 -- Ellipsoidal Solid/RConn1
  Trafo lower leg joint Right1/LConn1 -- Ankle/RConn1
  Trafo lower leg joint Right1/RConn1 -- Rotation/LConn1
  Ellipsoidal Solid/LConn1 -- Geom Foot/RConn1

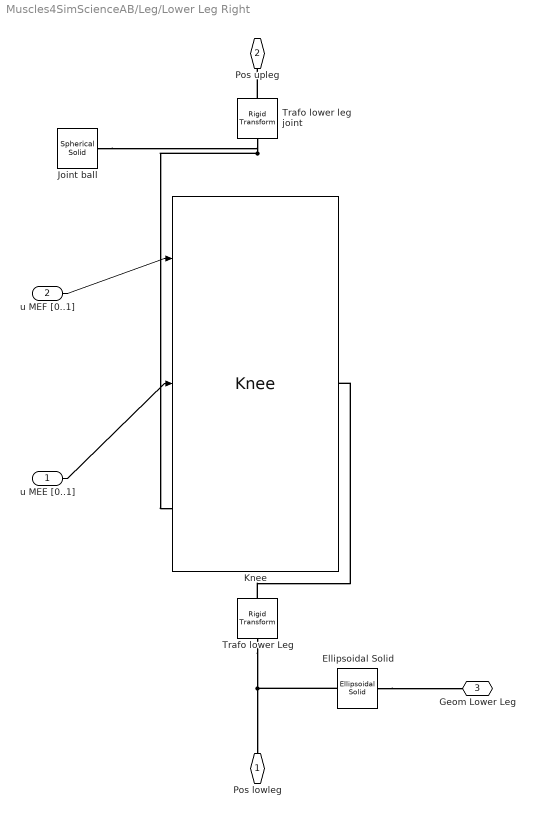
== system Muscles4SimScienceAB/Leg/Lower Leg Right ==
  u MEE [0..1] : Inport
  u MEF [0..1] : Inport  Port=2
  Ellipsoidal Solid : sm_lib/Body Elements/Ellipsoidal Solid  GraphicAmbientColor=[0.15 0.15 0.15 1.0]  BasedOnType=Density  CenterOfMass=sp.lowerleg  CenterOfMassUnits=m  GraphicDiffuseColor=lcolor  Density=1000  DensityUnits=kg/m^3  DoExposeReferenceFrame=on  EllipsoidRadii=size.lowerleg/2  EllipsoidRadiiUnits=m  GraphicEmissiveColor=[0.0 0.0 0.0 1.0]  ExportEntireGeometry=on  SerializedFrames=<Frames/>  MarkerShape=Sphere  MarkerSize=10  GraphicType=FromGeometry  InertiaType=Custom  Mass=weight.lowerleg  MassUnits=kg  MomentsOfInertia=[1 1 1]  MomentsOfInertiaUnits=kg*m^2  GraphicOpacity=1.0  ProductsOfInertia=[0 0 0]  ProductsOfInertiaUnits=kg*m^2  GraphicShininess=75  GraphicSpecularColor=[0.5 0.5 0.5 1.0]  GraphicVisPropType=SimpleVisualProperties
      settings: SourceProductBaseCode=MS
  Joint ball : sm_lib/Body Elements/Spherical Solid  GraphicAmbientColor=[0.15 0.15 0.15 1.0]  BasedOnType=Mass  CenterOfMass=[0 0 0]  CenterOfMassUnits=m  GraphicDiffuseColor=jcolor  Density=1000  DensityUnits=kg/m^3  DoExposeReferenceFrame=on  GraphicEmissiveColor=[0.0 0.0 0.0 1.0]  ExportEntireGeometry=off  SerializedExposedGeometries=<ExposedGeometries/>  SerializedFrames=<Frames/>  MarkerShape=Sphere  MarkerSize=10  GraphicType=FromGeometry  InertiaType=CalculateFromGeometry  Mass=0  MassUnits=kg  MomentsOfInertia=[1 1 1]  MomentsOfInertiaUnits=kg*m^2  GraphicOpacity=1.0  ProductsOfInertia=[0 0 0]  ProductsOfInertiaUnits=kg*m^2  GraphicShininess=75  GraphicSpecularColor=[0.5 0.5 0.5 1.0]  SphereRadius=size.jointballs  SphereRadiusUnits=m  GraphicVisPropType=SimpleVisualProperties
  Knee : $bdroot/Knee  maxlim=maxlim.knee  minlim=minlim.knee  stiffness=stiffness.knee  damping=damping.knee
  Trafo lower Leg : sm_lib/Frames and Transforms/Rigid Transform  TranslationMethod=Cartesian  TranslationStandardOffset=0  TranslationLengthUnit=m  TranslationStandardAxis=+Z  TranslationCartesianOffset=pos.lowerleg.item  TranslationROffset=0  TranslationROffsetUnits=m  TranslationZOffset=0  TranslationZOffsetUnits=m  TranslationThetaOffset=0  TranslationThetaOffsetUnits=deg  RotationMethod=None  RotationAngleUnits=deg  RotationStandardAxis=+Z  RotationAngle=0.0  RotationArbitraryAxis=[0 0 1]  FollAlignAxisA=+X  BaseAlignAxisA=+Y  FollAlignAxisB=+Y  BaseAlignAxisB=+Z  RotationSequenceAxes=FollowerAxes  RotationSequence=XYX  RotationSequenceAngles=[0 0 0]  RotationSequenceAnglesUnits=deg  RotationMatrix=[1 0 0; 0 1 0; 0 0 1]
  Trafo lower leg joint : sm_lib/Frames and Transforms/Rigid Transform  TranslationMethod=Cartesian  TranslationStandardOffset=0  TranslationLengthUnit=m  TranslationStandardAxis=+Z  TranslationCartesianOffset=pos.lowerleg.joint  TranslationROffset=0  TranslationROffsetUnits=m  TranslationZOffset=0  TranslationZOffsetUnits=m  TranslationThetaOffset=0  TranslationThetaOffsetUnits=deg  RotationMethod=None  RotationAngleUnits=deg  RotationStandardAxis=+Z  RotationAngle=0.0  RotationArbitraryAxis=[0 0 1]  FollAlignAxisA=+X  BaseAlignAxisA=+Y  FollAlignAxisB=+Y  BaseAlignAxisB=+Z  RotationSequenceAxes=FollowerAxes  RotationSequence=XYX  RotationSequenceAngles=[0 0 0]  RotationSequenceAnglesUnits=deg  RotationMatrix=[1 0 0; 0 1 0; 0 0 1]
  Pos lowleg : PMIOPort  Side=Left
  Pos upleg : PMIOPort  Port=2  Side=Right
  "Geom Lower Leg " : PMIOPort  Port=3  Side=Right
  wires:
  u MEE [0..1]/1 -> Knee/2
  u MEF [0..1]/1 -> Knee/1
  connections:
  Ellipsoidal Solid/LConn1 -- "Geom Lower Leg "/RConn1
  Trafo lower leg joint/LConn1 -- Pos upleg/RConn1
  Trafo lower leg joint/RConn1 -- Joint ball/RConn1 -- Knee/LConn1
  Trafo lower Leg/LConn1 -- Knee/RConn1
  Trafo lower Leg/RConn1 -- Ellipsoidal Solid/RConn1 -- Pos lowleg/RConn1

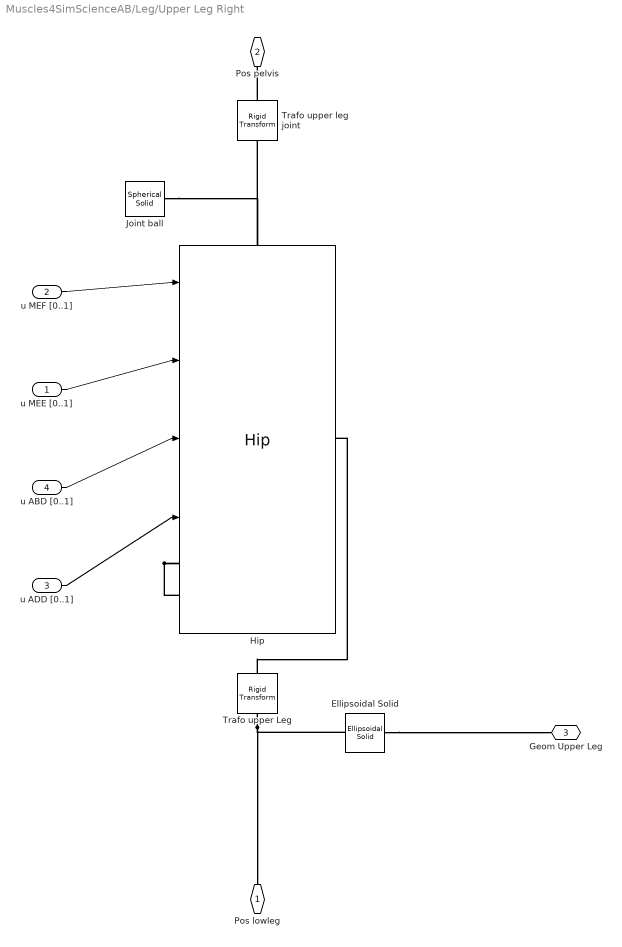
== system Muscles4SimScienceAB/Leg/Upper Leg Right ==
  u MEE [0..1] : Inport
  u MEF [0..1] : Inport  Port=2
  u ADD [0..1] : Inport  Port=3
  u ABD [0..1] : Inport  Port=4
  Ellipsoidal Solid : sm_lib/Body Elements/Ellipsoidal Solid  GraphicAmbientColor=[0.15 0.15 0.15 1.0]  BasedOnType=Density  CenterOfMass=[0 0 0]  CenterOfMassUnits=m  GraphicDiffuseColor=lcolor  Density=1000  DensityUnits=kg/m^3  DoExposeReferenceFrame=on  EllipsoidRadii=size.upperleg/2  EllipsoidRadiiUnits=m  GraphicEmissiveColor=[0.0 0.0 0.0 1.0]  ExportEntireGeometry=on  SerializedFrames=<Frames/>  MarkerShape=Sphere  MarkerSize=10  GraphicType=FromGeometry  InertiaType=CalculateFromGeometry  Mass=1  MassUnits=kg  MomentsOfInertia=[1 1 1]  MomentsOfInertiaUnits=kg*m^2  GraphicOpacity=1.0  ProductsOfInertia=[0 0 0]  ProductsOfInertiaUnits=kg*m^2  GraphicShininess=75  GraphicSpecularColor=[0.5 0.5 0.5 1.0]  GraphicVisPropType=SimpleVisualProperties
      settings: SourceProductBaseCode=MS
  Hip : $bdroot/Hip  minlim_x=0  maxlim_x=0  minlim_y=0  maxlim_y=0  stiffness=0  damping=0
  Joint ball : sm_lib/Body Elements/Spherical Solid  GraphicAmbientColor=[0.15 0.15 0.15 1.0]  BasedOnType=Mass  CenterOfMass=[0 0 0]  CenterOfMassUnits=m  GraphicDiffuseColor=jcolor  Density=1000  DensityUnits=kg/m^3  DoExposeReferenceFrame=on  GraphicEmissiveColor=[0.0 0.0 0.0 1.0]  ExportEntireGeometry=off  SerializedExposedGeometries=<ExposedGeometries/>  SerializedFrames=<Frames/>  MarkerShape=Sphere  MarkerSize=10  GraphicType=FromGeometry  InertiaType=CalculateFromGeometry  Mass=0  MassUnits=kg  MomentsOfInertia=[1 1 1]  MomentsOfInertiaUnits=kg*m^2  GraphicOpacity=1.0  ProductsOfInertia=[0 0 0]  ProductsOfInertiaUnits=kg*m^2  GraphicShininess=75  GraphicSpecularColor=[0.5 0.5 0.5 1.0]  SphereRadius=size.jointballs_hip  SphereRadiusUnits=m  GraphicVisPropType=SimpleVisualProperties
  Trafo upper Leg : sm_lib/Frames and Transforms/Rigid Transform  TranslationMethod=Cartesian  TranslationStandardOffset=0  TranslationLengthUnit=m  TranslationStandardAxis=+Z  TranslationCartesianOffset=pos.upperleg.item  TranslationROffset=0  TranslationROffsetUnits=m  TranslationZOffset=0  TranslationZOffsetUnits=m  TranslationThetaOffset=0  TranslationThetaOffsetUnits=deg  RotationMethod=None  RotationAngleUnits=deg  RotationStandardAxis=+Z  RotationAngle=0.0  RotationArbitraryAxis=[0 0 1]  FollAlignAxisA=+X  BaseAlignAxisA=+Y  FollAlignAxisB=+Y  BaseAlignAxisB=+Z  RotationSequenceAxes=FollowerAxes  RotationSequence=XYX  RotationSequenceAngles=[0 0 0]  RotationSequenceAnglesUnits=deg  RotationMatrix=[1 0 0; 0 1 0; 0 0 1]
  Trafo upper leg joint : sm_lib/Frames and Transforms/Rigid Transform  TranslationMethod=Cartesian  TranslationStandardOffset=0  TranslationLengthUnit=m  TranslationStandardAxis=+Z  TranslationCartesianOffset=pos.upperleg.joint  TranslationROffset=0  TranslationROffsetUnits=m  TranslationZOffset=0  TranslationZOffsetUnits=m  TranslationThetaOffset=0  TranslationThetaOffsetUnits=deg  RotationMethod=None  RotationAngleUnits=deg  RotationStandardAxis=+Z  RotationAngle=0.0  RotationArbitraryAxis=[0 0 1]  FollAlignAxisA=+X  BaseAlignAxisA=+Y  FollAlignAxisB=+Y  BaseAlignAxisB=+Z  RotationSequenceAxes=FollowerAxes  RotationSequence=XYX  RotationSequenceAngles=[0 0 0]  RotationSequenceAnglesUnits=deg  RotationMatrix=[1 0 0; 0 1 0; 0 0 1]
  Pos lowleg : PMIOPort  Side=Left
  Pos pelvis : PMIOPort  Port=2  Side=Right
  "Geom Upper Leg " : PMIOPort  Port=3  Side=Right
  wires:
  u MEF [0..1]/1 -> Hip/1
  u MEE [0..1]/1 -> Hip/2
  u ABD [0..1]/1 -> Hip/3
  u ADD [0..1]/1 -> Hip/4
  connections:
  Trafo upper Leg/RConn1 -- Ellipsoidal Solid/RConn1 -- Pos lowleg/RConn1
  Hip/LConn1 -- Trafo upper leg joint/RConn1 -- Joint ball/RConn1
  Ellipsoidal Solid/LConn1 -- "Geom Upper Leg "/RConn1
  Trafo upper leg joint/LConn1 -- Pos pelvis/RConn1
  Trafo upper Leg/LConn1 -- Hip/RConn1
